simulink library "AddOn_Lib_TTC580_CCP"  (R2021a)
settings: Solver=VariableStepAuto  StartTime=0.0  StopTime=10.0  RelTol=1e-3
PreLoadFcn:
  | addpath(genpath(fileparts(which('AddOn_Lib_TTC580_CCP'))));
  | try
  | addpath([fileparts(which('AddOn_Lib_TTC580_CCP')),'\..\CustomClasses']);
  | catch
  | warning('AddOn_Lib_TTC580: add path to CustomClasses manually');
  | end
undefined symbols (not defined in the file): IO_Blk_Lib_TTC500, MainDlg_basic, MainDlg_CCP_J1939_
(part 1 of 3)
settings Model: Creator=hokka  LastModifiedBy=hokka
settings SolverCC: AlgebraicLoopSolver=TrustRegion
settings DataIOCC: ReturnWorkspaceOutputs=off
settings DebuggingCC: SFMachineParentedDataDiag=warning  ArithmeticOperatorsInVariantConditions=warning
settings SFSimCC: SimUseLocalCustomCode=off  CustomCodeUndefinedFunction=UseInterfaceOnly
settings RTWCC: RTWUseLocalCustomCode=off

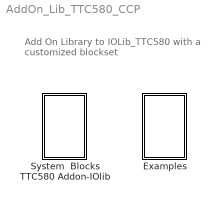
== system AddOn_Lib_TTC580_CCP ==
  note: Add On Library to IOLib_TTC580
      | with a customized blockset
  Examples : Subsystem
  System  Blocks TTC580 Addon-IOlib : Subsystem

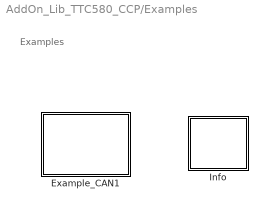
== system AddOn_Lib_TTC580_CCP/Examples ==
  note: Examples
  Example_CAN1 : Subsystem  mask{ble=0}
      settings: OpenFcn=|
      | sExampleName = 'Example_IOBlock_Library_CCP'; %without_extention
      | try
      | cd(fileparts(which(sExampleName)));
      | open_system(sExampleName);
      | catch
      | disp([sExampleName,' is not on MATLABPATH. Please check your installation of the IOLib. ']);
      | end
      mask Display: disp('Example using\nCCP CRO/DTO')
  Info : Subsystem  mask{bla=0}
      settings: OpenFcn=open('HowToUse_CCP_IOLib.pdf');
      mask Display: disp('Info\nCCP')
